simulink library "Communication"  (Simulink 7.4)
settings: Solver=ode45  StartTime=0.0  StopTime=10.0  RelTol=1e-3
PostLoadFcn:
  | load CommunicationBus.mat
(part 2 of 2)

== stateflow chart Communication/Convoy/convoy  ==
  settings: updateMethod=DISCRETE
  state simulation / [parallel]
    entry: state = 0;
    settings: executionOrder=2
    state convoy_handling [parallel]
      settings: executionOrder=1
      state no_convoy
        entry: coordinator = ID;
        entry: convoyMaxVelocity = NULL_DOUBLE;
        entry: convoyMaxBrake = NULL_DOUBLE;
        entry: convoyNormalBrake = NULL_DOUBLE;
        entry: convoyJoinVelocity = NULL_DOUBLE;
        entry: convoyJoinPosition = NULL_DOUBLE;
        entry: brakeDelay = NULL_DOUBLE;
        entry: following_shuttle = NULL_UINT8;
        entry: preceding_shuttle = NULL_UINT8;
        state reactingOnConvoyFormation
          state idle /
            entry: state[0] = 1;
          state waitingToRetry /
            entry: state[0] = 8;
          waitingToRetry  -> simulation.convoy_handling.no_convoy.reactingOnConvoyFormation.idle  : after(delay,wakeup)
        state waitForConvoyProperties /
          entry: state[0] = 3;
        state waitForConvoyApproval /
          entry: state[0] = 2;
        state decideOnConvoyJoining /
          entry: state[0] = 4;
        state waitForParams /
          entry: state[0] = 9;
        simulation.convoy_handling.no_convoy.reactingOnConvoyFormation.idle  -> waitForConvoyApproval  : [convoyUseful == 1]
            | {enqueue(EVT_CONVOY_REQUEST,NULL_DOUBLE,counterpart);
            |  enqueue(EVT_SHUTTLE_MAX_VELOCITY,maxVelocity,counterpart);
            |  enqueue(EVT_SHUTTLE_MAX_BRAKE,maxBrake,counterpart);
            |  enqueue(EVT_SHUTTLE_NORMAL_BRAKE,normalBrake,counterpart);}
        (default) -> simulation.convoy_handling.no_convoy.reactingOnConvoyFormation.idle 
        waitForConvoyApproval  -> waitForConvoyProperties  [order 3] : [checkQueue(EVT_CONVOY_APPROVAL,counterpart)]
            | {dequeue(EVT_CONVOY_APPROVAL,counterpart);}
        waitForConvoyApproval  -> simulation.convoy_handling.no_convoy.reactingOnConvoyFormation.idle  [order 2] : [checkQueue(EVT_CONVOY_DENIAL,counterpart)]
            | {dequeue(EVT_CONVOY_DENIAL,counterpart);}
        waitForConvoyProperties  -> decideOnConvoyJoining  : [checkQueue(EVT_CONVOY_MAX_VELOCITY,counterpart) && checkQueue(EVT_CONVOY_MAX_BRAKE,counterpart) && checkQueue(EVT_CONVOY_NORMAL_BRAKE,counterpart) && checkQueue(EVT_CONVOY_JOIN_VELOCITY,counterpart) && checkQueue(EVT_CONVOY_JOIN_POSITION,counterpart)]
            | {convoyMaxVelocity = dequeue(EVT_CONVOY_MAX_VELOCITY,counterpart);
            |  convoyMaxBrake = dequeue(EVT_CONVOY_MAX_BRAKE,counterpart);
            |  convoyNormalBrake = dequeue(EVT_CONVOY_NORMAL_BRAKE,counterpart);
            |  convoyJoinVelocity = dequeue(EVT_CONVOY_JOIN_VELOCITY,counterpart);
            |  convoyJoinPosition = dequeue(EVT_CONVOY_JOIN_POSITION,counterpart);}
        waitForConvoyApproval  -> simulation.convoy_handling.no_convoy.reactingOnConvoyFormation.idle  [order 1] : [checkQueue(EVT_SHUTTLE_NON_COORDINATOR,counterpart)]
            | {dequeue(EVT_SHUTTLE_NON_COORDINATOR,counterpart)}
        decideOnConvoyJoining  -> simulation.convoy_handling.no_convoy.reactingOnConvoyFormation.idle  [order 1] : [convoyUseful == 0]
            | {enqueue(EVT_CONVOY_REVOCATION,NULL_DOUBLE,counterpart);}
        decideOnConvoyJoining  -> waitingToRetry  [order 2] : [!in(coordination.coordinator.normal.idle)]
            | {enqueue(EVT_CONVOY_REVOCATION,NULL_DOUBLE,counterpart);
            | delay = randomDelay();}
        decideOnConvoyJoining  -> waitForParams  [order 3] : [convoyUseful == 1 && in(coordination.coordinator.normal.idle)]
            | {enqueue(EVT_CONVOY_AFFIRMATION,NULL_DOUBLE,counterpart);
            | send(enteredConvoy,coordination);
            | coordinator = counterpart}
        waitForParams  -> waitForParams  [order 2] : [checkQueue(EVT_CONVOY_FOLLOWING_SHUTTLE, coordinator)]
            | {following_shuttle = dequeue(EVT_CONVOY_FOLLOWING_SHUTTLE, coordinator);}
        waitForParams  -> waitForParams  [order 3] : [checkQueue(EVT_CONVOY_PRECEDING_SHUTTLE, coordinator)]
            | {preceding_shuttle = dequeue(EVT_CONVOY_PRECEDING_SHUTTLE, coordinator);}
      state convoy
        state reactingOnCoordinatorChange
          state idle /
            entry: state[0] = 5;
          state waitForConvoyExit /
            entry: state[0] = 6;
          (default) -> simulation.convoy_handling.convoy.reactingOnCoordinatorChange.idle 
          simulation.convoy_handling.convoy.reactingOnCoordinatorChange.idle  -> waitForConvoyExit  [order 4] : [convoyUseful == 0 && coordinator != ID]
              | {enqueue(EVT_CONVOY_LEAVE_REQUEST,NULL_DOUBLE,coordinator);
              | responder = coordinator;}
          waitForConvoyExit  -> simulation.convoy_handling.convoy.reactingOnCoordinatorChange.idle  [order 1] : [checkQueue(EVT_CONVOY_LEAVE_DENIAL,coordinator)]
              | {dequeue(EVT_CONVOY_LEAVE_DENIAL,coordinator);}
          waitForConvoyExit  -> simulation.convoy_handling.convoy.reactingOnCoordinatorChange.idle  [order 3] : [checkQueue(EVT_SHUTTLE_NON_COORDINATOR,responder)]
              | {dequeue(EVT_SHUTTLE_NON_COORDINATOR,responder)}
          simulation.convoy_handling.convoy.reactingOnCoordinatorChange.idle  -> simulation.convoy_handling.convoy.reactingOnCoordinatorChange.idle  [order 3] : adoptedCoordination
              | {coordinator = ID;}
          simulation.convoy_handling.convoy.reactingOnCoordinatorChange.idle  -> simulation.convoy_handling.convoy.reactingOnCoordinatorChange.idle  [order 2] : [checkQueue(EVT_CONVOY_FOLLOWING_SHUTTLE, coordinator)]
              | {following_shuttle = dequeue(EVT_CONVOY_FOLLOWING_SHUTTLE, coordinator);}
          simulation.convoy_handling.convoy.reactingOnCoordinatorChange.idle  -> simulation.convoy_handling.convoy.reactingOnCoordinatorChange.idle  [order 5] : [checkQueue(EVT_CONVOY_PRECEDING_SHUTTLE, coordinator)]
              | {preceding_shuttle = dequeue(EVT_CONVOY_PRECEDING_SHUTTLE, coordinator);}
          simulation.convoy_handling.convoy.reactingOnCoordinatorChange.idle  -> simulation.convoy_handling.convoy.reactingOnCoordinatorChange.idle  [order 6] : [checkQueue(EVT_CONVOY_MAX_VELOCITY,coordinator) && checkQueue(EVT_CONVOY_MAX_BRAKE,coordinator) && checkQueue(EVT_CONVOY_NORMAL_BRAKE,coordinator) && checkQueue(EVT_SHUTTLE_BRAKE_DELAY,coordinator)]
              | {convoyMaxVelocity = dequeue(EVT_CONVOY_MAX_VELOCITY,coordinator);
              | convoyMaxBrake = dequeue(EVT_CONVOY_MAX_BRAKE,coordinator);
              | convoyNormalBrake = dequeue(EVT_CONVOY_NORMAL_BRAKE,coordinator);
              | brakeDelay = dequeue(EVT_SHUTTLE_BRAKE_DELAY,coordinator);}
        state waitForCoordinatorChange /
          entry: state[0] = 7;
        (default) -> reactingOnCoordinatorChange
        (junction 115) -> (history) : {coordinator = getSender(EVT_CONVOY_COORDINATION_CHANGE);
            | dequeue(EVT_CONVOY_COORDINATION_CHANGE,coordinator)}
        reactingOnCoordinatorChange -> waitForCoordinatorChange  : [checkQueue(EVT_CONVOY_COORDINATION_ANNOUNCEMENT,NULL_UINT8)]
            | {enqueue(EVT_SHUTTLE_MAX_VELOCITY,maxVelocity,getSender(EVT_CONVOY_COORDINATION_ANNOUNCEMENT));
            |  enqueue(EVT_SHUTTLE_MAX_BRAKE,maxBrake,getSender(EVT_CONVOY_COORDINATION_ANNOUNCEMENT));
            |  enqueue(EVT_SHUTTLE_NORMAL_BRAKE,normalBrake,getSender(EVT_CONVOY_COORDINATION_ANNOUNCEMENT));
            |  dequeue(EVT_CONVOY_COORDINATION_ANNOUNCEMENT,getSender(EVT_CONVOY_COORDINATION_ANNOUNCEMENT));}
        waitForCoordinatorChange  -> (junction 116) : [checkQueue(EVT_CONVOY_COORDINATION_CHANGE,NULL_UINT8)]
        (junction 116) -> (junction 115) [order 1] : [coordinator != ID]
        (junction 116) -> (junction 115) [order 2] : [coordinator == ID && in(coordination.coordinator.waitingForCoordinationAdoption)]
            | {send(deliverCoordination,coordination)}
      (default) -> no_convoy
      reactingOnConvoyFormation -> convoy : convoyFormed
      simulation.convoy_handling.convoy.reactingOnCoordinatorChange.idle  -> no_convoy [order 1] : convoyDismissed
      waitForConvoyExit  -> no_convoy [order 2] : [checkQueue(EVT_CONVOY_LEAVE_APPROVAL,coordinator) && in(coordination.non_coordinator.idle)]
          | {dequeue(EVT_CONVOY_LEAVE_APPROVAL,coordinator);
          | send(leftConvoy,coordination)}
      waitForParams  -> simulation.convoy_handling.convoy.reactingOnCoordinatorChange.idle  [order 1] : [checkQueue(EVT_CONVOY_MAX_VELOCITY,coordinator) && checkQueue(EVT_CONVOY_MAX_BRAKE,coordinator) && checkQueue(EVT_CONVOY_NORMAL_BRAKE,coordinator) && checkQueue(EVT_SHUTTLE_BRAKE_DELAY,coordinator)]
          | {convoyMaxVelocity = dequeue(EVT_CONVOY_MAX_VELOCITY,coordinator);
          | convoyMaxBrake = dequeue(EVT_CONVOY_MAX_BRAKE,coordinator);
          | convoyNormalBrake = dequeue(EVT_CONVOY_NORMAL_BRAKE,coordinator);
          | brakeDelay = dequeue(EVT_SHUTTLE_BRAKE_DELAY,coordinator);}
    state coordination [parallel]
      settings: executionOrder=2
      state coordinator /
        entry: shuttles = NULL_UINT8;
        entry: shuttles_maxVelocity = NULL_DOUBLE;
        entry: shuttles_maxBrake = NULL_DOUBLE;
        entry: shuttles_normalBrake = NULL_DOUBLE;
        state normal
          state waitingForShuttleProperties /
            entry: state[1] = 2;
          state decidingOnConvoyExit /
            entry: state[1] = 8;
          state idle /
            entry: requester = NULL_UINT8;
            entry: ingest(ID, maxVelocity, maxBrake, normalBrake);
            entry: state[1] = 1;
          state decidingOnConvoyAccess /
            entry: state[1] = 3;
          state waitingForConvoyAffirmation /
            entry: state[1] = 4;
          state waitingToBroadcastConvoyProperties /
            entry: state[1] = 6;
          state waitingToNotifyDismissal /
            entry: state[1] = 7;
          state waitingToNotifyFormation /
            entry: state[1] = 5;
          (default) -> simulation.coordination.coordinator.normal.idle 
          simulation.coordination.coordinator.normal.idle  -> waitingForShuttleProperties  [order 2] : [checkQueue(EVT_CONVOY_REQUEST,NULL_UINT8)]
              | {requester = getSender(EVT_CONVOY_REQUEST);
              | dequeue(EVT_CONVOY_REQUEST,requester);}
          waitingForShuttleProperties  -> decidingOnConvoyAccess  : [checkQueue(EVT_SHUTTLE_MAX_VELOCITY,requester) && checkQueue(EVT_SHUTTLE_MAX_BRAKE,requester) && checkQueue(EVT_SHUTTLE_NORMAL_BRAKE,requester)]
              | {tmp_shuttleMaxVelocity=dequeue(EVT_SHUTTLE_MAX_VELOCITY,requester);
              | tmp_shuttleMaxBrake=dequeue(EVT_SHUTTLE_MAX_BRAKE,requester);
              | tmp_shuttleNormalBrake=dequeue(EVT_SHUTTLE_NORMAL_BRAKE,requester)}
          simulation.coordination.coordinator.normal.idle  -> decidingOnConvoyExit  [order 3] : [checkQueue(EVT_CONVOY_LEAVE_REQUEST,NULL_UINT8)]
              | {requester = getSender(EVT_CONVOY_LEAVE_REQUEST);
              | dequeue(EVT_CONVOY_LEAVE_REQUEST,requester)}
          decidingOnConvoyExit  -> (junction 121) [order 1] : [grantExit == 1]
              | {enqueue(EVT_CONVOY_LEAVE_APPROVAL,NULL_DOUBLE,requester);}
          decidingOnConvoyExit  -> simulation.coordination.coordinator.normal.idle  [order 2] : [grantExit == 0]
              | {enqueue(EVT_CONVOY_LEAVE_DENIAL,NULL_DOUBLE,requester)}
          decidingOnConvoyAccess  -> simulation.coordination.coordinator.normal.idle  [order 1] : [grantJoining == 0]
              | {enqueue(EVT_CONVOY_DENIAL,NULL_DOUBLE,requester);}
          waitingToBroadcastConvoyProperties  -> simulation.coordination.coordinator.normal.idle  : {propagateMaxVelocity();
              | propagateMaxBrake();
              | propagateNormalBrake();
              | propagateBrakeDelay();}
          waitingForConvoyAffirmation  -> simulation.coordination.coordinator.normal.idle  [order 1] : [checkQueue(EVT_CONVOY_REVOCATION,requester)]
              | {dequeue(EVT_CONVOY_REVOCATION,requester)}
          decidingOnConvoyAccess  -> (junction 117) [order 2] : [grantJoining == 1]
              | {enqueue(EVT_CONVOY_APPROVAL,NULL_DOUBLE,requester);
              |  enqueue(EVT_CONVOY_JOIN_VELOCITY,joinVelocity,requester);
              |  enqueue(EVT_CONVOY_JOIN_POSITION,joinPosition,requester);}
          waitingToNotifyDismissal  -> waitingToBroadcastConvoyProperties  [order 1] : [shuttleCount() > 1]
          waitingToNotifyFormation  -> waitingToBroadcastConvoyProperties  [order 2] : [shuttleCount() == 2 && in(convoy_handling.no_convoy.reactingOnConvoyFormation)]
              | {send(convoyFormed,convoy_handling)}
          waitingForConvoyAffirmation  -> (junction 120) [order 2] : [checkQueue(EVT_CONVOY_AFFIRMATION,requester)]
              | {ingest(requester, tmp_shuttleMaxVelocity, tmp_shuttleMaxBrake, tmp_shuttleNormalBrake);
              | dequeue(EVT_CONVOY_AFFIRMATION,requester);
              | tmp_shuttleMaxVelocity = NULL_DOUBLE; tmp_shuttleMaxBrake = NULL_DOUBLE;
              | tmp_shuttleNormalBrake = NULL_DOUBLE;}
          waitingToNotifyDismissal  -> waitingToBroadcastConvoyProperties  [order 2] : [shuttleCount() == 1 && in(convoy_handling.convoy.reactingOnCoordinatorChange.idle)]
              | {send(convoyDismissed,convoy_handling)}
          waitingToNotifyFormation  -> waitingToBroadcastConvoyProperties  [order 1] : [shuttleCount() > 2]
          (junction 117) -> (junction 118) [order 1] : [computeMaxBrake()<tmp_shuttleMaxBrake]
              | {enqueue(EVT_CONVOY_MAX_BRAKE,computeMaxBrake(),requester);}
          (junction 117) -> (junction 118) [order 2] : [computeMaxBrake()>=tmp_shuttleMaxBrake]
              | {enqueue(EVT_CONVOY_MAX_BRAKE,tmp_shuttleMaxBrake,requester);}
          (junction 118) -> (junction 119) [order 1] : [computeNormalBrake()<tmp_shuttleNormalBrake]
              | {enqueue(EVT_CONVOY_NORMAL_BRAKE,computeNormalBrake(),requester);}
          (junction 118) -> (junction 119) [order 2] : [computeNormalBrake()>=tmp_shuttleNormalBrake]
              | {enqueue(EVT_CONVOY_NORMAL_BRAKE,tmp_shuttleNormalBrake,requester);}
          (junction 119) -> waitingForConvoyAffirmation  [order 1] : [computeMaxVelocity()<tmp_shuttleMaxVelocity]
              | {enqueue(EVT_CONVOY_MAX_VELOCITY,computeMaxVelocity(),requester);}
          (junction 119) -> waitingForConvoyAffirmation  [order 2] : [computeMaxVelocity()>=tmp_shuttleMaxVelocity]
              | {enqueue(EVT_CONVOY_MAX_VELOCITY,tmp_shuttleMaxVelocity,requester);}
          (junction 120) -> (junction 123) [order 3] : [getPrecedingShuttle(requester) ~= ID]
              | {enqueue(EVT_CONVOY_FOLLOWING_SHUTTLE, requester, getPrecedingShuttle(requester));}
          (junction 120) -> (junction 123) [order 1] : [getPrecedingShuttle(requester) == ID]
              | {following_shuttle = requester;}
          (junction 124) -> waitingToNotifyDismissal  : {release(requester);}
          (junction 121) -> (junction 122) [order 1] : [getPrecedingShuttle(requester) ~= ID]
              | {enqueue(EVT_CONVOY_FOLLOWING_SHUTTLE, getFollowingShuttle(requester), getPrecedingShuttle(requester));}
          (junction 121) -> (junction 122) [order 3] : [getPrecedingShuttle(requester) == ID]
              | {following_shuttle = getFollowingShuttle(requester);}
          (junction 120) -> (junction 123) [order 2] : [getPrecedingShuttle(requester) == 0]
          (junction 122) -> (junction 124) [order 2] : [getFollowingShuttle(requester)==0]
          (junction 122) -> (junction 124) [order 3] : [getFollowingShuttle(requester) == ID]
              | {preceding_shuttle = getPrecedingShuttle(requester);}
          (junction 123) -> waitingToNotifyFormation  : {enqueue(EVT_CONVOY_PRECEDING_SHUTTLE, getPrecedingShuttle(requester), requester);}
          (junction 121) -> (junction 122) [order 2] : [getPrecedingShuttle(requester) == 0]
          (junction 122) -> (junction 124) [order 1] : [getFollowingShuttle(requester) ~= ID]
              | {enqueue(EVT_CONVOY_PRECEDING_SHUTTLE, getPrecedingShuttle(requester), getFollowingShuttle(requester));}
        state waitingForCoordinationAdoption /
          entry: state[1] = 10;
        state waitingForCoordinationApproval /
          entry: state[1] = 9;
        (default) -> normal
        simulation.coordination.coordinator.normal.idle  -> waitingForCoordinationApproval  [order 4] : [coordinationUseful == 0 && isMember(counterpart) && counterpart != ID]
            | {enqueue(EVT_CONVOY_COORDINATION_REQUEST,array2decimal(shuttles),counterpart);}
        waitingForCoordinationApproval  -> normal [order 1] : [checkQueue(EVT_CONVOY_COORDINATION_DENIAL,counterpart)]
            | {dequeue(EVT_CONVOY_COORDINATION_DENIAL,counterpart);}
        waitingForCoordinationApproval  -> waitingForCoordinationAdoption  [order 2] : [checkQueue(EVT_CONVOY_COORDINATION_APPROVAL,counterpart)]
            | {dequeue(EVT_CONVOY_COORDINATION_APPROVAL,counterpart);}
      state non_coordinator
        state waitToAnnounceCoordination /
          entry: state[1] = 14;
        state idle /
          entry: requester = NULL_UINT8;
          entry: state[1] = 11;
          entry: shuttles = NULL_UINT8;
        state waitToAdoptCoordination /
          entry: state[1] = 16;
        state decidingOnCoordinationAdoption /
          entry: state[1] = 13;
        state wairForShuttleProperties /
          entry: state[1] = 15;
        state waitForShuttleProperties /
          entry: state[1] = 12;
        (default) -> simulation.coordination.non_coordinator.idle 
        simulation.coordination.non_coordinator.idle  -> simulation.coordination.non_coordinator.idle  [order 4] : [checkQueue(EVT_CONVOY_LEAVE_REQUEST,NULL_UINT8)]
            | {requester = getSender(EVT_CONVOY_LEAVE_REQUEST);
            | dequeue(EVT_CONVOY_LEAVE_REQUEST,requester);
            | enqueue(EVT_SHUTTLE_NON_COORDINATOR,NULL_DOUBLE,requester);}
        waitToAnnounceCoordination  -> wairForShuttleProperties  : {ingest(ID, maxVelocity, maxBrake, normalBrake);
            | multiEnqueue(EVT_CONVOY_COORDINATION_ANNOUNCEMENT,NULL_DOUBLE); tmp_shuttle=1;
            | tmp_shuttleMaxVelocity = NULL_DOUBLE; tmp_shuttleMaxBrake = NULL_DOUBLE;
            | tmp_shuttleNormalBrake = NULL_DOUBLE;}
        decidingOnCoordinationAdoption  -> waitToAnnounceCoordination  [order 2] : [coordinationUseful == 1]
            | {enqueue(EVT_CONVOY_COORDINATION_APPROVAL,NULL_DOUBLE,requester);}
        simulation.coordination.non_coordinator.idle  -> decidingOnCoordinationAdoption  [order 2] : [checkQueue(EVT_CONVOY_COORDINATION_REQUEST,NULL_DOUBLE)]
            | {requester = getSender(EVT_CONVOY_COORDINATION_REQUEST);
            | shuttles = decimal2array(dequeue(EVT_CONVOY_COORDINATION_REQUEST,requester));
            | shuttles_maxVelocity = NULL_DOUBLE; shuttles_maxBrake = NULL_DOUBLE; shuttles_normalBrake = NULL_DOUBLE;}
        decidingOnCoordinationAdoption  -> simulation.coordination.non_coordinator.idle  [order 1] : [coordinationUseful == 0]
            | {enqueue(EVT_CONVOY_COORDINATION_DENIAL,NULL_DOUBLE,requester)}
        waitForShuttleProperties  -> simulation.coordination.non_coordinator.idle  : [checkQueue(EVT_SHUTTLE_MAX_VELOCITY,requester) && checkQueue(EVT_SHUTTLE_MAX_BRAKE,requester) && checkQueue(EVT_SHUTTLE_NORMAL_BRAKE,requester)]
            | {dequeue(EVT_CONVOY_REQUEST,requester);
            | dequeue(EVT_SHUTTLE_MAX_VELOCITY,requester);
            | dequeue(EVT_SHUTTLE_MAX_BRAKE,requester);
            | dequeue(EVT_SHUTTLE_NORMAL_BRAKE,requester);
            | enqueue(EVT_SHUTTLE_NON_COORDINATOR,NULL_DOUBLE,requester);}
        simulation.coordination.non_coordinator.idle  -> waitForShuttleProperties  [order 3] : [checkQueue(EVT_CONVOY_REQUEST,NULL_UINT8)]
            | {requester = getSender(EVT_CONVOY_REQUEST);}
        wairForShuttleProperties  -> waitToAdoptCoordination  [order 6] : [checkShuttleProperties()]
            | {propagateMaxVelocity(); propagateMaxBrake();
            | propagateNormalBrake(); propagateBrakeDelay();}
        wairForShuttleProperties  -> wairForShuttleProperties  [order 2] : [checkQueue(EVT_SHUTTLE_MAX_VELOCITY, shuttles[tmp_shuttle])]
            | {tmp_shuttleMaxVelocity = dequeue(EVT_SHUTTLE_MAX_VELOCITY, shuttles[tmp_shuttle]);}
        wairForShuttleProperties  -> wairForShuttleProperties  [order 3] : [checkQueue(EVT_SHUTTLE_MAX_BRAKE, shuttles[tmp_shuttle])]
            | {tmp_shuttleMaxBrake = dequeue(EVT_SHUTTLE_MAX_BRAKE, shuttles[tmp_shuttle]);}
        wairForShuttleProperties  -> wairForShuttleProperties  [order 4] : [checkQueue(EVT_SHUTTLE_NORMAL_BRAKE, shuttles[tmp_shuttle])]
            | {tmp_shuttleNormalBrake = dequeue(EVT_SHUTTLE_NORMAL_BRAKE, shuttles[tmp_shuttle]);}
        wairForShuttleProperties  -> wairForShuttleProperties  [order 5] : [tmp_shuttleMaxVelocity ~= NULL_DOUBLE  && tmp_shuttleMaxBrake ~= NULL_DOUBLE && tmp_shuttleNormalBrake ~= NULL_DOUBLE]
            | {ingest(shuttles[tmp_shuttle], tmp_shuttleMaxVelocity, tmp_shuttleMaxBrake, tmp_shuttleNormalBrake);
            | tmp_shuttle++; tmp_shuttleMaxVelocity = NULL_DOUBLE; tmp_shuttleMaxBrake = NULL_DOUBLE; tmp_shuttleNormalBrake = NULL_DOUBLE;}
        wairForShuttleProperties  -> wairForShuttleProperties  [order 1] : [(shuttles[tmp_shuttle] == NULL_UINT8 || shuttles[tmp_shuttle] == ID) && tmp_shuttle < SHUTTLE_COUNT]
            | {tmp_shuttle++;}
      simulation.coordination.coordinator.normal.idle  -> non_coordinator [order 1] : enteredConvoy
      waitingForCoordinationAdoption  -> non_coordinator : deliverCoordination
      simulation.coordination.non_coordinator.idle  -> coordinator  [order 1] : leftConvoy
      waitToAdoptCoordination  -> coordinator  : [in(convoy_handling.convoy.reactingOnCoordinatorChange.idle)]
          | {multiEnqueue(EVT_CONVOY_COORDINATION_CHANGE,NULL_DOUBLE);
          | send(adoptedCoordination,convoy_handling);}
    simulation  -> simulation  : [reset]
        | {writeEventQueueIn = NULL_UINT8;
        | writeEventQueueOut = NULL_UINT8;
        | writeParamQueueIn = NULL_DOUBLE;
        | writeParamQueueOut = NULL_DOUBLE}
    (default) -> coordinator 
  state data_read [parallel]
    settings: executionOrder=1
    data_read -> data_read : wakeup
        | {read;
        | writeEventQueueIn = readEventQueueIn;
        | writeEventQueueOut = readEventQueueOut;
        | writeParamQueueIn = readParamQueueIn;
        | writeParamQueueOut = readParamQueueOut;}
  state data_write [parallel]
    settings: executionOrder=3
    data_write -> data_write : wakeup
        | {write;}
    (default) -> ? : wakeup
        | {write;}
  data: id function_input uint8; member function_output boolean; array function_output uint8 size=5; dec function_input double; array function_input uint8 size=5; dec function_output double; event function_input uint8; parameter function_output double; sender function_input uint8; event function_input uint8; available function_output boolean; sender function_input uint8; event function_input uint8; parameter function_input double; receiver function_input uint8; r function_output double; x local uint8; count function_output double; id function_input uint8; event function_input uint8; sender function_output uint8; event function_input uint8; event function_input uint8; available function_output boolean; event function_input uint8; parameter function_input double; id function_input uint8; maxV function_input double; maxB function_input double; normalB function_input double; allReceived function_output boolean; minMaxVelocity function_output double; minNormalBrake function_output double; minMaxBrake function_output double; id function_input uint8; pre function_output uint8; id function_input uint8; post function_output uint8; commerror input boolean; state output uint8 size=2; coordinationUseful input boolean; joinPosition input double; buffer_overrun output boolean; convoyJoinPosition output double; convoyJoinVelocity output double; joinVelocity input double; maxVelocity input double; maxBrake input double; normalBrake input double; convoyBrakeDelay input double size=SHUTTLE_COUNT; convoyMaxVelocity output double; convoyMaxBrake output double; convoyNormalBrake output double; brakeDelay output double; readEventQueueIn input uint8 size=[10,2]; readParamQueueIn input double size=10; readEventQueueOut input uint8 size=[10,2]; readParamQueueOut input double size=10; writeEventQueueIn output uint8 size=[10,2]; writeParamQueueIn output double size=10; writeEventQueueOut output uint8 size=[10,2]; writeParamQueueOut output double size=10; following_shuttle output uint8; NULL_DOUBLE constant double; NULL_UINT8 constant uint8; counterpart input double; grantJoining input double; grantExit input double; requester local uint8; coordinator output uint8; EVT_COMMERROR_RESUME_ACK constant uint8 =1; EVT_CONVOY_AFFIRMATION constant uint8 =2; EVT_CONVOY_APPROVAL constant uint8 =3; EVT_CONVOY_COORDINATION_ANNOUNCEMENT constant uint8 =4; EVT_CONVOY_COORDINATION_APPROVAL constant uint8 =5; EVT_CONVOY_COORDINATION_CHANGE constant uint8 =6; EVT_CONVOY_COORDINATION_DENIAL constant uint8 =7; EVT_CONVOY_COORDINATION_REQUEST constant uint8 =8; EVT_CONVOY_DENIAL constant uint8 =9; EVT_CONVOY_JOIN_POSITION constant uint8 =10; EVT_CONVOY_JOIN_VELOCITY constant uint8 =11; EVT_CONVOY_LEAVE_APPROVAL constant uint8 =12; EVT_CONVOY_LEAVE_DENIAL constant uint8 =13; EVT_CONVOY_LEAVE_REQUEST constant uint8 =14; EVT_CONVOY_MAX_BRAKE constant uint8 =15; EVT_CONVOY_MAX_VELOCITY constant uint8 =16; EVT_CONVOY_NORMAL_BRAKE constant uint8 =17; EVT_CONVOY_REQUEST constant uint8 =18; EVT_CONVOY_REVOCATION constant uint8 =19; EVT_SHUTTLE_BRAKE_DELAY constant uint8 =20; EVT_SHUTTLE_MAX_BRAKE constant uint8 =21; EVT_SHUTTLE_MAX_VELOCITY constant uint8 =22; EVT_SHUTTLE_NORMAL_BRAKE constant uint8 =23; shuttles output uint8 size=[SHUTTLE_COUNT,1]; convoyUseful input boolean; ID input uint8; EVT_SHUTTLE_NON_COORDINATOR constant uint8 =24; reset input boolean; responder local uint8; delay local double; SHUTTLE_COUNT constant double =5; shuttles_maxVelocity local double size=SHUTTLE_COUNT; shuttles_maxBrake local double size=SHUTTLE_COUNT; shuttles_normalBrake local double size=SHUTTLE_COUNT; tmp_shuttleMaxVelocity local double; tmp_shuttleMaxBrake local double; tmp_shuttleNormalBrake local double; tmp_shuttle local uint8 =1; EVT_CONVOY_FOLLOWING_SHUTTLE constant uint8 =25; EVT_CONVOY_PRECEDING_SHUTTLE constant uint8 =26; preceding_shuttle output uint8
  events: write output FUNCTION_CALL_EVENT; read output FUNCTION_CALL_EVENT; enteredConvoy local EITHER_EDGE_EVENT; leftConvoy local EITHER_EDGE_EVENT; deliverCoordination local EITHER_EDGE_EVENT; adoptedCoordination local EITHER_EDGE_EVENT; convoyFormed local EITHER_EDGE_EVENT; convoyDismissed local EITHER_EDGE_EVENT
  function propagateBrakeDelay:
    | function propagateBrakeDelay    
    | 
    | i = 1;
    | for j = 0:SHUTTLE_COUNT-1
    |     if shuttles(SHUTTLE_COUNT-j) ~= NULL_UINT8     
    |         if shuttles(SHUTTLE_COUNT-j) ~= ID
    |             enqueue(EVT_SHUTTLE_BRAKE_DELAY,convoyBrakeDelay(i),shuttles(SHUTTLE_COUNT-j));
    |         else
    |             brakeDelay = convoyBrakeDelay(i);
    |         end
    |         i = i+1;
    |     end
    | end
  function member = isMember(id):
    | function member = isMember(id)
    | 
    | for i = 1:SHUTTLE_COUNT
    |     if shuttles(i) == id 
    |         member = true;
    |         return
    |     end
    | end
    | member = false;
  function array = decimal2array(dec):
    | function array = decimal2array(dec)
    | 
    | array = [NULL_UINT8; NULL_UINT8; NULL_UINT8; NULL_UINT8; NULL_UINT8;];
    | 
    | for i = 0:SHUTTLE_COUNT-1
    |     array(SHUTTLE_COUNT-i) = mod(dec,10);
    |     dec = floor(dec/10);
    | end
  function dec = array2decimal(array):
    | function dec = array2decimal(array)
    | 
    | dec = 0;
    | 
    | for i = 0:SHUTTLE_COUNT-1
    |     dec = dec + cast(array(SHUTTLE_COUNT-i),'double')*power(10,i);
    | end
  function parameter = dequeue(event,sender):
    | function parameter = dequeue(event,sender)
    | 
    | parameter = NULL_DOUBLE;
    | for i = 1:10
    |     if writeEventQueueIn(i) == event
    |         if writeEventQueueIn(i+10) == sender
    |             parameter = writeParamQueueIn(i);
    |             for j = i:9
    |                 writeEventQueueIn(j) = writeEventQueueIn(j+1);
    |                 writeEventQueueIn(j+10) = writeEventQueueIn(j+11);
    |                 writeParamQueueIn(j) = writeParamQueueIn(j+1);
    |             end
    |             writeEventQueueIn(10) = NULL_UINT8;
    |             writeEventQueueIn(20) = NULL_UINT8;
    |             writeParamQueueIn(10) = NULL_DOUBLE;
    |             return
    |         end
    |     end
    | end
  function available = checkQueue(event,sender):
    | function available = checkQueue(event,sender)
    | 
    | for i = 1:10
    |     if writeEventQueueIn(i) == event
    |         if writeEventQueueIn(i+10) == sender || sender == NULL_UINT8
    |             available = true;
    |             return
    |         end    
    |     end
    | end
    | available = false;
  function enqueue(event,parameter,receiver):
    | function enqueue(event,parameter,receiver)
    | 
    | for i = 1:10
    |     if writeEventQueueOut(i) == NULL_UINT8
    |         writeEventQueueOut(i) = event;
    |         writeEventQueueOut(i+10) = receiver;
    |         writeParamQueueOut(i) = parameter;
    |         buffer_overrun = false;
    |         return
    |     end
    | end    
    | buffer_overrun = true;
  function r = randomDelay:
    | function r = randomDelay()
    | 
    | if delay == 0 || delay == 1
    |     delay = cast(ID,'double')+1;
    | end    
    | delay = mod(delay*delay,100);
    | r = delay;
  function count = shuttleCount:
    | function count = shuttleCount
    | 
    | count = 0;
    | for i = 1:SHUTTLE_COUNT
    |     if shuttles(i) ~= NULL_UINT8
    |         count = count+1;
    |     end
    | end
  function release(id):
    | function release(id)    
    | 
    | for i=1:SHUTTLE_COUNT
    |     if shuttles(i) == id
    |         shuttles(i) = NULL_UINT8;
    |         shuttles_maxVelocity(i) = NULL_DOUBLE;
    |         shuttles_maxBrake(i) = NULL_DOUBLE;
    |         shuttles_normalBrake(i) = NULL_DOUBLE;
    |         for j=i:SHUTTLE_COUNT-1
    |             shuttles(j) = shuttles(j+1);
    |             shuttles_maxVelocity(j) = shuttles_maxVelocity(j+1);
    |             shuttles_maxBrake(j) = shuttles_maxBrake(j+1);
    |             shuttles_normalBrake(j) = shuttles_normalBrake(j+1);
    |         end    
    |         return
    |     end
    | end
  function sender = getSender(event):
    | function sender = getSender(event)
    | 
    | for i = 1:10
    |     if writeEventQueueIn(i) == event
    |         sender = writeEventQueueIn(i+10);
    |         return
    |     end
    | end
    | sender = NULL_UINT8;
  function multiDequeue(event):
    | function multiDequeue(event)
    | 
    | for i = 1:SHUTTLE_COUNT
    |     if shuttles(i) ~= NULL_UINT8 && shuttles(i) ~= ID 
    |         dequeue(event,cast(shuttles(i),'uint8'));
    |     end    
    | end
  function available = multiCheckQueue(event):
    | function available = multiCheckQueue(event)
    | 
    | for i = 1:SHUTTLE_COUNT
    |     if shuttles(i) ~= NULL_UINT8 && shuttles(i) ~= ID && checkQueue(event,cast(shuttles(i),'uint8')) == false
    |         available = false;
    |         return
    |     end
    | end
    | available = true;
  function multiEnqueue(event,parameter):
    | function multiEnqueue(event,parameter)
    | 
    | for i = 1:SHUTTLE_COUNT
    |     if shuttles(i) ~= NULL_UINT8 && shuttles(i) ~= ID
    |         enqueue(event,parameter,cast(shuttles(i),'uint8'));
    |     end    
    | end
  function ingest(id, maxV, maxB, normalB):
    | function ingest(id, maxV, maxB, normalB)
    | 
    | for i = 1:SHUTTLE_COUNT
    |     if shuttles(i) == id 
    |         shuttles_maxVelocity(i) = maxV;
    |         shuttles_maxBrake(i) = maxB;
    |         shuttles_normalBrake(i) = normalB;
    |         return
    |     end
    | end
    | 
    | if SHUTTLE_COUNT == shuttleCount()
    |     buffer_overrun = true;
    |     return
    | end
    | 
    | for i=1:SHUTTLE_COUNT
    |     if shuttles(i) == NULL_UINT8
    |         shuttles(i) = id;
    |         shuttles_maxVelocity(i) = maxV;
    |         shuttles_maxBrake(i) = maxB;
    |         shuttles_normalBrake(i) = normalB;
    |         return
    |     end
    | end
  function propagateMaxVelocity:
    | function propagateMaxVelocity    
    | 
    | minMaxVelocity = computeMaxVelocity();
    |     
    | for i = 1:SHUTTLE_COUNT
    |     if shuttles(i) ~= NULL_UINT8     
    |         if shuttles(i) ~= ID
    |             enqueue(EVT_CONVOY_MAX_VELOCITY,minMaxVelocity,shuttles(i));
    |         else
    |             convoyMaxVelocity = minMaxVelocity;
    |         end
    |     end
    | end
  function propagateMaxBrake:
    | function propagateMaxBrake    
    | 
    | minMaxBrake = computeMaxBrake();
    |     
    | for i = 1:SHUTTLE_COUNT
    |     if shuttles(i) ~= NULL_UINT8     
    |         if shuttles(i) ~= ID
    |             enqueue(EVT_CONVOY_MAX_BRAKE,minMaxBrake,shuttles(i));
    |         else
    |             convoyMaxBrake = minMaxBrake;
    |         end
    |     end
    | end
  function propagateNormalBrake:
    | function propagateNormalBrake    
    | 
    | minNormalBrake = computeNormalBrake();
    | 
    | for i = 1:SHUTTLE_COUNT
    |     if shuttles(i) ~= NULL_UINT8     
    |         if shuttles(i) ~= ID
    |             enqueue(EVT_CONVOY_NORMAL_BRAKE,minNormalBrake,shuttles(i));
    |         else
    |             convoyNormalBrake = minNormalBrake;
    |         end
    |     end
    | end
  function allReceived = checkShuttleProperties:
    | function allReceived = checkShuttleProperties
    | 
    | allReceived = true;
    | 
    | for i = 1:SHUTTLE_COUNT
    |     if shuttles(i) ~= NULL_UINT8
    |         received = (shuttles_maxVelocity(i) ~= NULL_DOUBLE) && (shuttles_maxBrake(i) ~= NULL_DOUBLE) && (shuttles_normalBrake(i) ~= NULL_DOUBLE);
    |         if (~received)
    |             allReceived = false;
    |             return
    |         end
    |     end
    | end
  function minMaxVelocity = computeMaxVelocity:
    | function minMaxVelocity = computeMaxVelocity    
    | 
    | minMaxVelocity = shuttles_maxVelocity(1);
    | 
    | for i=2:SHUTTLE_COUNT
    |     if ((shuttles(i) ~= NULL_DOUBLE && shuttles_maxVelocity(i) < minMaxVelocity) || minMaxVelocity==NULL_DOUBLE)
    |         minMaxVelocity = shuttles_maxVelocity(i);
    |     end
    | end
  function minNormalBrake = computeNormalBrake:
    | function minNormalBrake = computeNormalBrake    
    | 
    | minNormalBrake = shuttles_normalBrake(1);
    | 
    | for i=2:SHUTTLE_COUNT
    |     if ((shuttles(i) ~= NULL_DOUBLE && shuttles_normalBrake(i) < normalBrake) || minNormalBrake == NULL_DOUBLE)
    |         minNormalBrake = shuttles_normalBrake(i);
    |     end
    | end
  function minMaxBrake = computeMaxBrake:
    | function minMaxBrake = computeMaxBrake    
    | 
    | minMaxBrake = shuttles_maxBrake(1);
    | 
    | for i=2:SHUTTLE_COUNT
    |     if ((shuttles(i) ~= NULL_DOUBLE && shuttles_maxBrake(i) < minMaxBrake) || minMaxBrake == NULL_DOUBLE)
    |         minMaxBrake = shuttles_maxBrake(i);
    |     end
    | end
  function pre = getPrecedingShuttle(id):
    | function pre = getPrecedingShuttle(id)
    | 
    | pre = uint8(0); % id is first shuttle
    | 
    | for i = 1:SHUTTLE_COUNT
    |     if shuttles(i) == id
    |         if (i ~= 1) % id is not first shuttle
    |           pre = shuttles(i-1);
    |           return
    |         else
    |             pre = uint8(0); % id is first shuttle
    |             return
    |         end
    |     end
    | end
  function post = getFollowingShuttle(id):
    | function post = getFollowingShuttle(id)
    | 
    | post = uint8(0); % id is last shuttle
    | 
    | for i = 1:SHUTTLE_COUNT
    |     if shuttles(i) == id
    |         if (i ~= SHUTTLE_COUNT) % id is not last shuttle
    |           post = shuttles(i+1);
    |           return
    |         else
    |             post = uint8(0); % id is last shuttle
    |             return
    |         end
    |     end
    | end
